simulink model "Posture_Regulation_NO_Singularity"  (R2022b)
settings: Solver=FixedStepAuto  StartTime=0.0  StopTime=10.0  MaxStep=0.1  RelTol=1e-3
undefined symbols (not defined in the file): theta_f, unicycle, x_f, y_f
libraries: simulink_extras x2
settings Model: Creator=Musta  LastModifiedBy=mustacchim

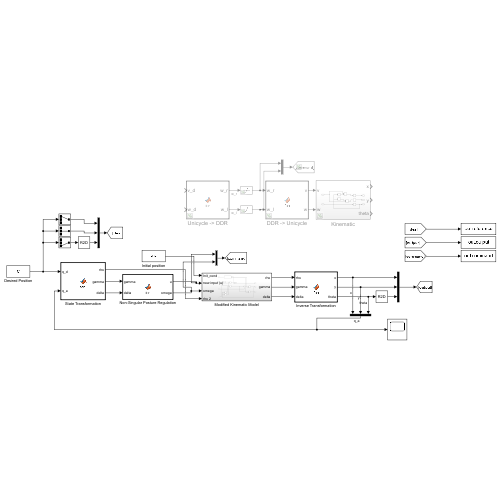
[thumbnail: Simulink's stored preview of the top-level diagram]
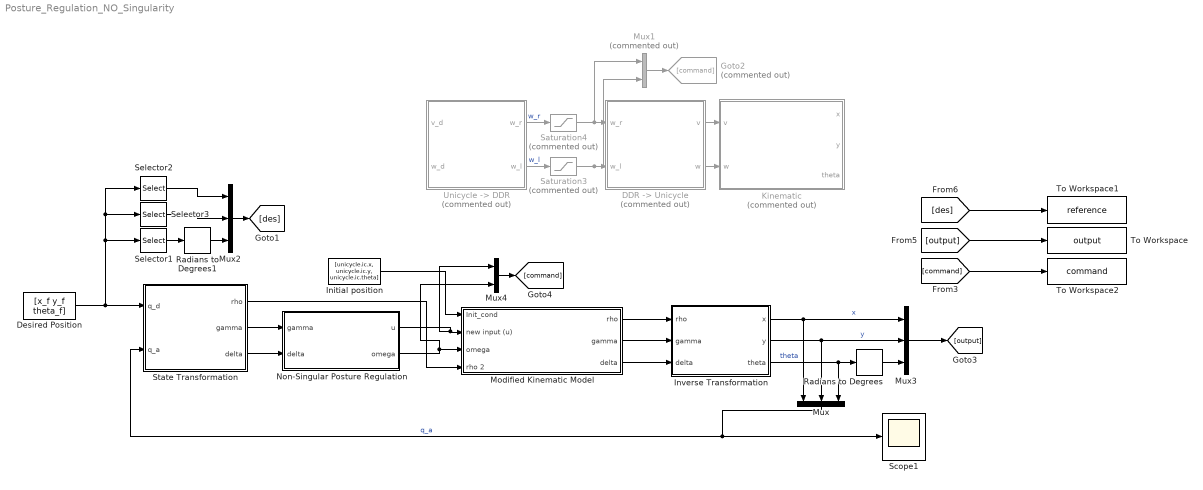
== system Posture_Regulation_NO_Singularity ==
  " DDR -> Unicycle " : MATLAB Function  Commented=on  TreatAsAtomicUnit=on
  Desired Position : Constant  Value=[x_f y_f theta_f]
  Goto2 : Goto  Commented=on  GotoTag=command
  Initial position : Constant  Value=[unicycle.ic.x, unicycle.ic.y, unicycle.ic.theta]
  Inverse Transformation : MATLAB Function  TreatAsAtomicUnit=on
  Kinematic : Subsystem  Commented=on
  Modified Kinematic Model : Subsystem
  Mux : Mux  Inputs=3
  Mux1 : Mux  Commented=on  Inputs=2
  Mux2 : Mux  Inputs=3
  Mux3 : Mux  Inputs=3
  Mux4 : Mux  Inputs=2
  Non-Singular Posture Regulation : MATLAB Function  TreatAsAtomicUnit=on
  Radians to Degrees : simulink_extras/Transformations/Radians to Degrees
  Radians to Degrees1 : simulink_extras/Transformations/Radians to Degrees
  Saturation3 : Saturate  Commented=on  UpperLimit=unicycle.omegaWheelMax  LowerLimit=unicycle.omegaWheelMin
  Saturation4 : Saturate  Commented=on  UpperLimit=unicycle.omegaWheelMax  LowerLimit=unicycle.omegaWheelMin
  Scope1 : Scope
  Selector1 : Selector  InputPortWidth=3  IndexOptions=Index vector (dialog)  Indices=3  OutputSizes=1
  Selector2 : Selector  InputPortWidth=3  IndexOptions=Index vector (dialog)  Indices=1  OutputSizes=1
  Selector3 : Selector  InputPortWidth=3  IndexOptions=Index vector (dialog)  Indices=2  OutputSizes=1
  State Transformation : MATLAB Function  TreatAsAtomicUnit=on
  To Workspace : ToWorkspace  VariableName=output  SaveFormat=Structure With Time  SampleTime=-1
  To Workspace1 : ToWorkspace  VariableName=reference  SaveFormat=Structure With Time  SampleTime=-1
  To Workspace2 : ToWorkspace  VariableName=command  SaveFormat=Structure With Time  SampleTime=-1
  "Unicycle -> DDR" : MATLAB Function  Commented=on  TreatAsAtomicUnit=on
  wires:
  [command] -> To Workspace2/1
  [des] -> To Workspace1/1
  [output] -> To Workspace/1
  Selector2/1 -> Mux2/1
  Mux/1 -> Scope1/1, State Transformation/2(q_a)  "q_a"
  Selector3/1 -> Mux2/2
  Inverse Transformation/1(x) -> Mux/1, Mux3/1  "x"
  Desired Position/1 -> Selector2/1, Selector3/1, Selector1/1, State Transformation/1(q_d)
  Inverse Transformation/3(theta) -> Mux/3, Radians to Degrees/1  "theta"
  Radians to Degrees/1 -> Mux3/3
  Inverse Transformation/2(y) -> Mux3/2, Mux/2  "y"
  Modified Kinematic Model/3(delta) -> Inverse Transformation/3(delta)
  Mux2/1 -> [des]
  State Transformation/1(rho) -> Modified Kinematic Model/4(rho 2)
  Radians to Degrees1/1 -> Mux2/3
  Selector1/1 -> Radians to Degrees1/1
  Modified Kinematic Model/1(rho) -> Inverse Transformation/1(rho)
  Mux4/1 -> [command]
  Modified Kinematic Model/2(gamma) -> Inverse Transformation/2(gamma)
  State Transformation/3(delta) -> Non-Singular Posture Regulation/2(delta)
  Initial position/1 -> Modified Kinematic Model/1(Init_cond)
  Non-Singular Posture Regulation/1(u) -> Modified Kinematic Model/2(new input (u)), Mux4/1
  Mux3/1 -> [output]
  Non-Singular Posture Regulation/2(omega) -> Mux4/2, Modified Kinematic Model/3(omega)
  State Transformation/2(gamma) -> Non-Singular Posture Regulation/1(gamma)
  "Unicycle -> DDR"/2(w_l) -> Saturation3/1  "w_l"
  " DDR -> Unicycle "/1(v) -> Kinematic/1(v)
  "Unicycle -> DDR"/1(w_r) -> Saturation4/1  "w_r"
  Mux1/1 -> Goto2/1
  Saturation4/1 -> Mux1/1, " DDR -> Unicycle "/1(w_r)
  Saturation3/1 -> Mux1/2, " DDR -> Unicycle "/2(w_l)
  " DDR -> Unicycle "/2(w) -> Kinematic/2(w)

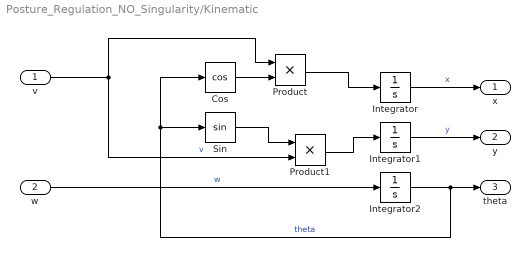
== system Posture_Regulation_NO_Singularity/Kinematic ==
  v : Inport
  w : Inport  Port=2
  Cos : Trigonometry  Operator=cos
  Integrator : Integrator  InitialCondition=unicycle.ic.x
  Integrator1 : Integrator  InitialCondition=unicycle.ic.y
  Integrator2 : Integrator  InitialCondition=unicycle.ic.theta
  Product : Product
  Product1 : Product
  Sin : Trigonometry
  x : Outport
  y : Outport  Port=2
  theta : Outport  Port=3
  wires:
  w/1 -> Integrator2/1  "w"
  Product/1 -> Integrator/1
  v/1 -> Product/1, Product1/2  "v"
  Cos/1 -> Product/2
  Integrator1/1 -> y/1  "y"
  Integrator/1 -> x/1  "x"
  Integrator2/1 -> Cos/1, Sin/1, theta/1  "theta"
  Product1/1 -> Integrator1/1
  Sin/1 -> Product1/1

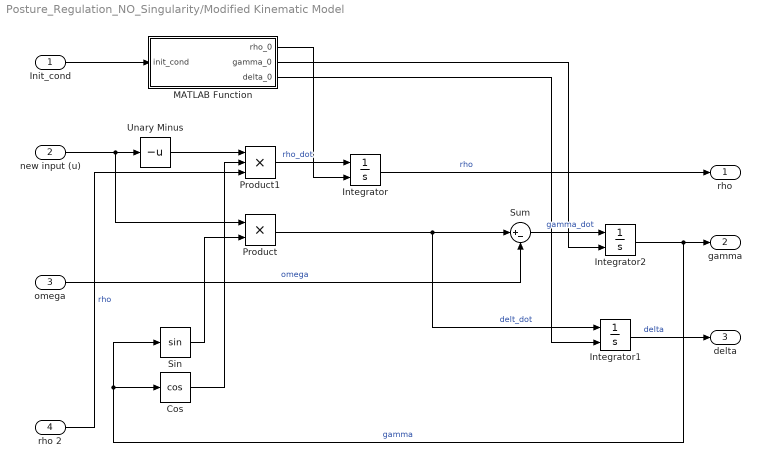
== system Posture_Regulation_NO_Singularity/Modified Kinematic Model ==
  Init_cond : Inport
  new input (u) : Inport  Port=2
  omega : Inport  Port=3
  rho 2 : Inport  Port=4
  Cos : Trigonometry  Operator=cos
  Integrator : Integrator  InitialConditionSource=external  InitialCondition=-10
  Integrator1 : Integrator  InitialConditionSource=external
  Integrator2 : Integrator  InitialConditionSource=external
  MATLAB Function : MATLAB Function  TreatAsAtomicUnit=on
  Product : Product
  Product1 : Product  Inputs=3
  Sin : Trigonometry
  Sum : Sum  Inputs=|+-
  Unary Minus : UnaryMinus
  rho : Outport
  gamma : Outport  Port=2
  delta : Outport  Port=3
  wires:
  Sum/1 -> Integrator2/1  "gamma_dot"
  Cos/1 -> Product1/2
  Unary Minus/1 -> Product1/1
  new input (u)/1 -> Product/1, Unary Minus/1
  Product1/1 -> Integrator/1  "rho_dot"
  Integrator/1 -> rho/1  "rho"
  Sin/1 -> Product/2
  Product/1 -> Sum/1, Integrator1/1  "delt_dot"
  omega/1 -> Sum/2  "omega"
  Integrator2/1 -> gamma/1, Cos/1, Sin/1  "gamma"
  Integrator1/1 -> delta/1  "delta"
  rho 2/1 -> Product1/3  "rho"
  Init_cond/1 -> MATLAB Function/1(init_cond)
  MATLAB Function/2(gamma_0) -> Integrator2/2
  MATLAB Function/3(delta_0) -> Integrator1/2
  MATLAB Function/1(rho_0) -> Integrator/2

== matlab function Posture_Regulation_NO_Singularity/ DDR -> Unicycle  ==
  data: w_r input; v output; w_l input; w output
function [v, w] = fcn(w_r, w_l)

    %#codegen
    coder.extrinsic('evalin')
    d = 0;                  % Needed in order to set variable class correctly
    r = 0;                  % Needed in order to set variable class correctly
    d = evalin('base','unicycle.d'); % Read value from workspace
    r = evalin('base','unicycle.r'); % Read value from workspace

    v = r*(w_r + w_l)/2; % rad/s
    w = r*(w_r - w_l)/d; % rad/s

end

== matlab function Posture_Regulation_NO_Singularity/Non-Singular Posture Regulation ==
  data: u output; omega output; gamma input; delta input
function [u,omega] = fcn(gamma,delta)

    %#codegen
    coder.extrinsic('evalin')
    k1 = 0;                  % Needed in order to set variable class correctly
    k2 = 0;                  % Needed in order to set variable class correctly
    k3 = 0;                  % Needed in order to set variable class correctly
    k1 = evalin('base','k1'); % Read value from workspace
    k2 = evalin('base','k2'); % Read value from workspace
    k3 = evalin('base','k3'); % Read value from workspace

    u = k1 * cos(gamma);
    omega = k2 * gamma + (k1 * sin(gamma)*cos(gamma)/gamma * (gamma + k3 * delta));

end

== matlab function Posture_Regulation_NO_Singularity/State Transformation ==
  data: q_d input; rho output; q_a input; gamma output; delta output
function [rho,gamma,delta] = fcn(q_d, q_a)

    e_x = q_d(1) - q_a(1);
    e_y = q_d(2) - q_a(2);
    e_theta = q_d(3) - q_a(3);
    
    rho = sqrt(e_x^2 + e_y^2);
    gamma = mod(atan2(e_y,e_x),2*pi) - q_a(3);
    delta = gamma - e_theta;

end

== matlab function Posture_Regulation_NO_Singularity/Inverse Transformation ==
  data: x output; rho input; y output; gamma input; delta input; theta output
function [x,y,theta] = fcn(rho,gamma,delta)

    x = - rho * cos(delta);
    y = - rho * sin(delta);
    theta = delta - gamma;
    
end

== matlab function Posture_Regulation_NO_Singularity/Modified Kinematic Model/MATLAB Function ==
  data: init_cond input; rho_0 output; gamma_0 output; delta_0 output
function [rho_0, gamma_0, delta_0] = fcn(init_cond)

x_0 = init_cond(1);
y_0 = init_cond(2);
theta_0 = init_cond(3);


rho_0 = sqrt(x_0^2 + y_0^2);
gamma_0 = atan2(y_0,x_0) - theta_0 + pi;
delta_0 = gamma_0 + theta_0;

== matlab function Posture_Regulation_NO_Singularity/Unicycle -> DDR ==
  data: v_d input; w_r output; w_d input; w_l output
function [w_r, w_l] = fcn(v_d, w_d)

    %#codegen
    coder.extrinsic('evalin')
    d = 0;                  % Needed in order to set variable class correctly
    r = 0;                  % Needed in order to set variable class correctly
    d = evalin('base','unicycle.d'); % Read value from workspace
    r = evalin('base','unicycle.r'); % Read value from workspace

    w_r = ((2 * v_d) + (w_d * d)) / (2 * r);
    w_l = ((2 * v_d) - (w_d * d)) / (2 * r);

end
